simulink model "zlinear_pid"  (R2019a)
settings: Solver=FixedStepAuto  StartTime=0.0  StopTime=100  FixedStep=1e-5  RelTol=1e-3
values from neighbouring files (symbols this model uses):
  g = 9.81    [dron.m]
  Ixx = 0.02276    [dron.m]
  Iyy = Ixx    (= 0.02276)    [dron.m]
  Izz = 0.03132    [dron.m]
  m = 1    [dron.m]
settings Model: Creator=alber  LastModifiedBy=alber
settings DataIOCC: ReturnWorkspaceOutputs=off

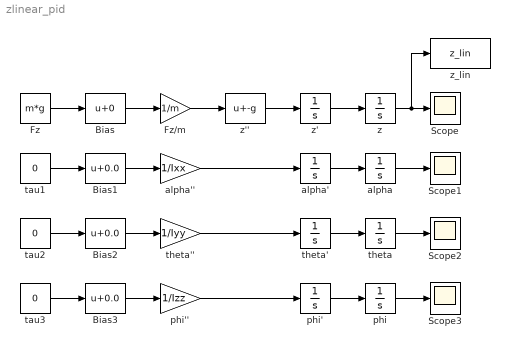
== system zlinear_pid ==
  Bias : Bias
  Bias1 : Bias  Bias=0.0
  Bias2 : Bias  Bias=0.0
  Bias3 : Bias  Bias=0.0
  Fz : Constant  Value=m*g
  Fz/m : Gain  Gain=1/m
  Scope{,1..3} (4 alike) : Scope
  alpha : Integrator
  alpha' : Integrator
  alpha'' : Gain  Gain=1/Ixx
  phi : Integrator
  phi' : Integrator
  phi'' : Gain  Gain=1/Izz
  tau1 : Constant  Value=0
  tau2 : Constant  Value=0
  tau3 : Constant  Value=0
  theta : Integrator
  theta' : Integrator
  theta'' : Gain  Gain=1/Iyy
  z : Integrator  InitialCondition=1
  z' : Integrator
  z'' : Bias  Bias=-g
  z_lin : ToWorkspace  VariableName=z_lin  SampleTime=1e-5
  wires:
  Fz/m/1 -> z''/1
  z''/1 -> z'/1
  z'/1 -> z/1
  z/1 -> z_lin/1, Scope/1
  tau1/1 -> Bias1/1
  alpha/1 -> Scope1/1
  alpha'/1 -> alpha/1
  alpha''/1 -> alpha'/1
  theta''/1 -> theta'/1
  theta'/1 -> theta/1
  theta/1 -> Scope2/1
  tau2/1 -> Bias2/1
  tau3/1 -> Bias3/1
  phi/1 -> Scope3/1
  phi'/1 -> phi/1
  phi''/1 -> phi'/1
  Fz/1 -> Bias/1
  Bias/1 -> Fz/m/1
  Bias1/1 -> alpha''/1
  Bias2/1 -> theta''/1
  Bias3/1 -> phi''/1
